simulink model "que8"  (R2020b)
settings: Solver=VariableStepAuto  StartTime=0.0  StopTime=10.0  RelTol=1e-3
settings Model: Creator=ANUJA  LastModifiedBy=ANUJA

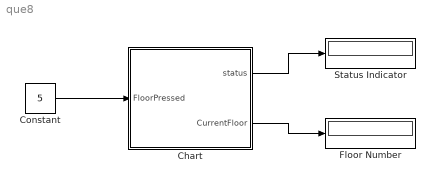
== system que8 ==
  Chart : Stateflow chart  TreatAsAtomicUnit=on
  Constant : Constant  Value=5
  Floor Number : Display
  Status Indicator : Display
  wires:
  Chart/2(CurrentFloor) -> Floor Number/1
  Constant/1 -> Chart/1(FloorPressed)
  Chart/1(status) -> Status Indicator/1

== stateflow chart que8/Chart ==
  state LiftOperation
    entry:
    status=0;
    state LiftFunctionOn [parallel]
      entry:
      status=1;
      settings: executionOrder=1
      state GroundFloor
        entry:
        status=1;
        during:
        CurrentFloor=0;
        FloorCheck(CurrentFloor);
        exit:
        status=0;
      state FirstFloor
        entry:
        status=1;
        during:
        CurrentFloor=1;
        FloorCheck(CurrentFloor);
        exit:
        status=0
      state SecondFloor
        entry:
        status=1;
        during:
        CurrentFloor=2;
        FloorCheck(CurrentFloor);
        exit:
        status=0;
      state ThirdFloor
        entry:
        status=1;
        during:
        CurrentFloor=3;
        FloorCheck(CurrentFloor);
        exit:
        status=0;
      state FourthFloor
        entry:
        status=1
        during:
        CurrentFloor=4;
        FloorCheck(CurrentFloor);
        exit:
        status=0;
      state FifthFloor
        entry:
        status=1;
        during:
        CurrentFloor=5;
        FloorCheck(CurrentFloor);
        exit:
        status=0;
      (default) -> GroundFloor
      GroundFloor -> FirstFloor : up
      FirstFloor -> GroundFloor [order 2] : down
      FirstFloor -> SecondFloor [order 1] : up
      SecondFloor -> FirstFloor [order 2] : down
      SecondFloor -> ThirdFloor [order 1] : up
      ThirdFloor -> SecondFloor [order 2] : down
      ThirdFloor -> FourthFloor [order 1] : up
      FourthFloor -> ThirdFloor [order 2] : down
      FourthFloor -> FifthFloor [order 1] : up
      FifthFloor -> FourthFloor : down
    state LiftFunctionOff [parallel]
      entry:
      status=0;
      settings: executionOrder=2
  state FloorCheck(Floor) [function]
    (default) -> (junction 83)
    (junction 83) -> (junction 86) [order 3] : [FloorPressed<Floor]
        | {send(down);
        | disp('GoingDown');}
    (junction 83) -> (junction 88) [order 1] : [FloorPressed>Floor]
        | {send(up);
        | disp('GoingUp');}
    (junction 83) -> (junction 85) [order 2] : [FloorPressed==Floor]
        | {disp('Current Floor');}
  (default) -> LiftOperation
  data: Floor function_input; status output; CurrentFloor output; FloorPressed input
  events: down local RISING_EDGE_EVENT; up local RISING_EDGE_EVENT
